simulink model "LB01B05"  (R2022b)
settings: Solver=ode45  StartTime=0.0  StopTime=20.0  MaxStep=0.01  RelTol=1e-3
settings Model: Creator=Andrey  LastModifiedBy=Andrey

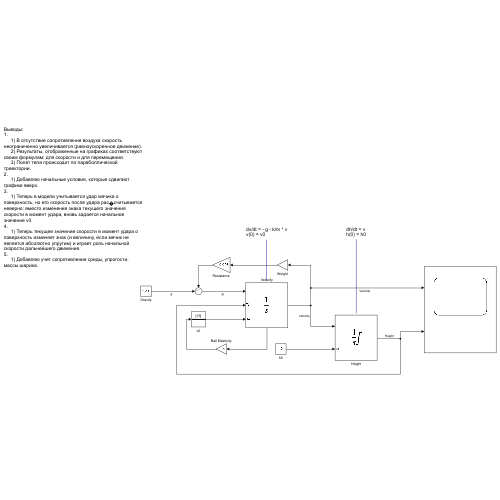
[thumbnail: Simulink's stored preview of the top-level diagram]
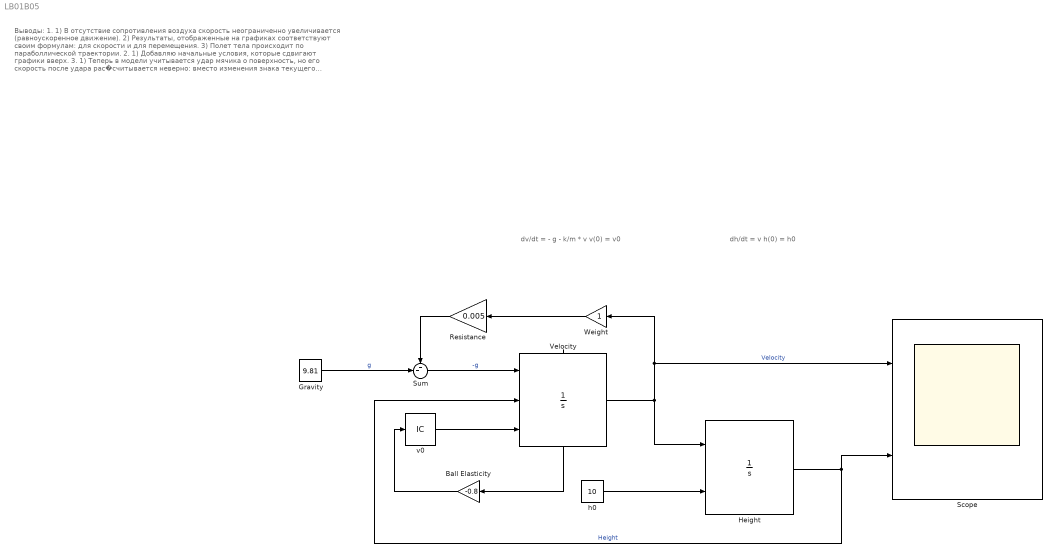
== system LB01B05 ==
  note: Выводы:
      | 1.
      | 1) В отсутствие сопротивления воздуха скорость неограниченно увеличивается (равноускоренное движение).
      | 2) Результаты, отображенные на графиках соответствуют своим формулам: для скорости и для перемещения.
      | 3) Полет тела происходит по параболлической траектории.
      | 2.
      | 1) Добавляю начальные условия, которые сдвигают графики вверх.
      | 3.
      | 1) Теперь в модели учитывается удар мячика о поверхность, но его скорость после удара рас�считывается неверно: вместо изменения знака текущего значения скорости в момент удара, вновь задается начальное значение v0.
      | 4.
      | 1) Теперь текущее значение скорости в момент удара о поверхность изменяет знак (и величину, если мячик не является абсолютно упругим) и играет роль начальной скорости дальнейшего движения.
      | 5.
      | 1) Добавляю учет сопротивления среды, упрогости, массы шарика.
  note: dh/dt = v
      | h(0) = h0
  note: dv/dt = - g - k/m * v
      | v(0) = v0
  Ball Elasticity : Gain  Gain=-0.8
  Gravity : Constant  Value=9.81
  Height : Integrator  InitialConditionSource=external  LimitOutput=on  LowerSaturationLimit=0
  Resistance : Gain  Gain=0.005
  Scope : Scope  NumInputPorts=2
  Sum : Sum  Inputs=--|
  Velocity : Integrator  ExternalReset=falling  InitialConditionSource=external  InitialCondition=1  ShowStatePort=on
  Weight : Gain
  h0 : Constant  Value=10
  v0 : InitialCondition  Value=15
  wires:
  Gravity/1 -> Sum/2  "g"
  Sum/1 -> Velocity/1  "-g"
  Velocity/1 -> Weight/1, Scope/1, Height/1  "Velocity"
  Height/1 -> Scope/2, Velocity/2  "Height"
  v0/1 -> Velocity/3
  h0/1 -> Height/2
  Velocity/State -> Ball Elasticity/1
  Ball Elasticity/1 -> v0/1
  Resistance/1 -> Sum/1
  Weight/1 -> Resistance/1
